simulink model "Sim_power_pedmap"  (R2025b)
settings: Solver=VariableStepAuto  StartTime=0.0  StopTime=15  RelTol=1e-3
undefined symbols (not defined in the file): LOCKED_FD_DAMP, LOCKED_FD_K, LOCKED_FD_OPT, M_DIFF_FD_TABLE, R_EFF_F_FD, R_EFF_R_FD, R_GEAR_FD
libraries: Solver_SF x1, simulink x1
settings Model: Creator=YNTM  LastModifiedBy=mayuan
settings RTWCC: GPUComputeCapability=3.5

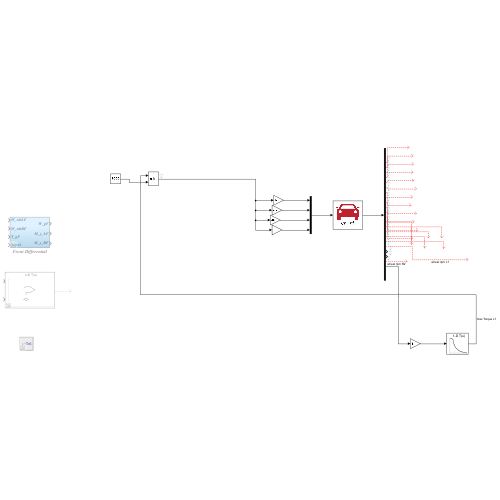
[thumbnail: Simulink's stored preview of the top-level diagram]
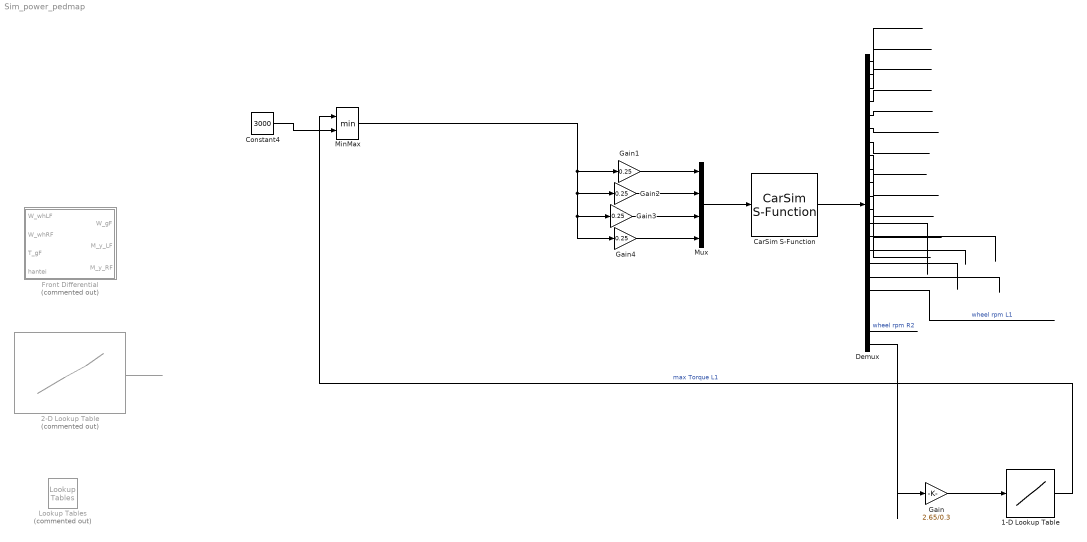
== system Sim_power_pedmap ==
  1-D Lookup Table : Lookup_n-D  NumberOfTableDimensions=1  BreakpointsForDimension1=[0, 50, 100, 150, 200, 250, 300, 350, 400, 450, 600].*3  Table=[3050, 3050, 2894.255, 1921.936, 1438.702, 1149.149, 956.489, 819.17, 717.149, 647.339, 477]  InternalRulePriority=Speed  RndMeth=Simplest
  2-D Lookup Table : Lookup_n-D  Commented=on  BreakpointsForDimension1=[0,5,15,20,25,30,40,50,60,70,80,90,100]  BreakpointsForDimension2=[0,7,10,20,30,40,50,60,70,80,100,120,140,160,180,200,220]  Table=|  InternalRulePriority=Speed  RndMeth=Simplest
      | [
      |     [0, 0, 0, 0, 0, 0, 0, 0, 0, 0, 0, 0, 0, 0, 0, 0, 0],
      |     [350, 350, 212, 104, 44, 22, 15, 15, 15, 15, 15, 15, 15, 15, 15, 15, 15],
      |     [765, 765, 641, 282, 149, 56, 100, 100, 100, 100, 100, 100, 100, 100, 100, 100, 100],
      |     [950, 950, 850, 621, 477, 354, 232, 200, 200, 200, 200, 200, 200, 200, 200, 200, 200],
      |     [1134, 1134, 1059, 959, 805, 652, 449, 300, 300, 300, 300, 300, 300, 300, 300, 300, 300],
      |     [1613, 1613, 1557, 1482, 1366, 1215, 1024, 846, 742, 656, 537, 463, 416, 398, 378, 362, 350],
      |     [2092, 2092, 2054, 2004, 1927, 1777, 1599, 1391, 1184, 1012, 774, 626, 532, 495, 455, 423, 400],
      |     [3049, 3049, 3049, 3049, 3049, 2902, 2749, 2482, 2068, 1724, 1247, 951, 763, 690, 610, 546, 500],
      |     [3752, 3752, 3752, 3752, 3751, 3629, 3484, 3235, 2850, 2524, 1978, 1598, 1329, 1173, 992, 867, 766],
      |     [4454, 4454, 4454, 4454, 4454, 4357, 4219, 3988, 3631, 3323, 2710, 2245, 1895, 1657, 1374, 1189, 1033],
      |     [5157, 5157, 5157, 5157, 5156, 5084, 4954, 4741, 4413, 4123, 3441, 2892, 2461, 2140, 1756, 1510, 1299],
      |     [5860, 5860, 5860, 5859, 5859, 5811, 5689, 5494, 5195, 4923, 4172, 3539, 3027, 2623, 2137, 1832, 1565],
      |     [6563, 6563, 6562, 6562, 6561, 6539, 6424, 6247, 5976, 5722, 4903, 4187, 3593, 3106, 2519, 2153, 1832],
      |     [7265, 7265, 7265, 7264, 7264, 7266, 7159, 7000, 6758, 6522, 5635, 4834, 4158, 3590, 2901, 2475, 2098]
      | ]
      settings: InputPortMap=u0,u1
  CarSim S-Function : Solver_SF/CarSim S-Function  Priority=1  SIMFILE=simfile.sim  Run_RTs=off  vs_state_ind=Run  StopMode_ind=Vehicle Model
  Constant4 : Constant  Value=3000
  Demux : Demux  Outputs=22
  "Front Differential " : Subsystem  Commented=on
  Gain : Gain  Gain=2.65/0.3
  Gain{1..4} (4 alike) : Gain  Gain=0.25
  Lookup Tables : simulink/Lookup Tables  Commented=on  SystemSampleTime=-1  VariantActivationTime=update diagram  EmptyChoice=off  PassThrough=off  PassThroughVariantControl=(default)  EmptyChoiceVariantControl=(default)  AllowFlexibleInterface=on  Latency=0  AutoFrameSizeCalculation=off
  MinMax : MinMax  Inputs=2
  Mux : Mux
  wires:
  MinMax/1 -> Gain4/1, Gain3/1, Gain2/1, Gain1/1
  Mux/1 -> CarSim S-Function/1
  CarSim S-Function/1 -> Demux/1
  Demux/1 -> ?
  Demux/2 -> ?
  Demux/3 -> ?
  Demux/4 -> ?
  Demux/5 -> ?
  Demux/6 -> ?
  Demux/7 -> ?
  Demux/8 -> ?
  Demux/9 -> ?
  Demux/10 -> ?
  Demux/11 -> ?
  Demux/12 -> ?
  Demux/13 -> ?
  Demux/14 -> ?
  Demux/15 -> ?
  Demux/16 -> ?
  Demux/17 -> ?
  2-D Lookup Table/1 -> ?
  Demux/18 -> ?  "wheel rpm L1"
  Demux/21 -> ?  "wheel rpm R2"
  1-D Lookup Table/1 -> MinMax/1  "max Torque L1"
  Constant4/1 -> MinMax/2
  Demux/22 -> Gain/1
  Gain/1 -> 1-D Lookup Table/1
  Gain1/1 -> Mux/1
  Gain2/1 -> Mux/2
  Gain3/1 -> Mux/3
  Gain4/1 -> Mux/4

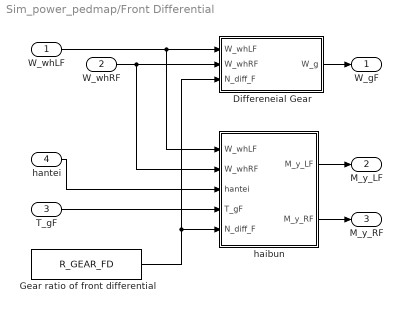
== system Sim_power_pedmap/Front Differential  ==
  W_whLF : Inport
  W_whRF : Inport  Port=2
  T_gF : Inport  Port=3
  hantei : Inport  Port=4
  Differeneial Gear : Subsystem
  Gear ratio of front differential : Constant  Value=R_GEAR_FD
  haibun : Subsystem
  W_gF : Outport
  M_y_LF : Outport  Port=2
  M_y_RF : Outport  Port=3
  wires:
  haibun/2(M_y_RF) -> M_y_RF/1
  haibun/1(M_y_LF) -> M_y_LF/1
  W_whRF/1 -> Differeneial Gear/2(W_whRF), haibun/2(W_whRF)
  W_whLF/1 -> Differeneial Gear/1(W_whLF), haibun/1(W_whLF)
  Gear ratio of front differential/1 -> haibun/5(N_diff_F), Differeneial Gear/3(N_diff_F)
  Differeneial Gear/1(W_g) -> W_gF/1
  T_gF/1 -> haibun/4(T_gF)
  hantei/1 -> haibun/3(hantei)

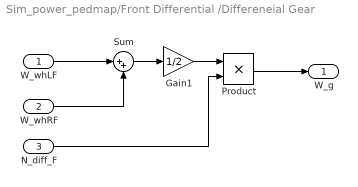
== system Sim_power_pedmap/Front Differential /Differeneial Gear ==
  W_whLF : Inport
  W_whRF : Inport  Port=2
  N_diff_F : Inport  Port=3
  Gain1 : Gain  Gain=1/2  SaturateOnIntegerOverflow=on  OutDataTypeStr=Inherit: Same as input  ParamDataTypeStr=Inherit: Same as input
  Product : Product  InputSameDT=on  SaturateOnIntegerOverflow=on  OutDataTypeStr=Inherit: Same as first input
  Sum : Sum  Inputs=|++  InputSameDT=on  SaturateOnIntegerOverflow=on  OutDataTypeStr=Inherit: Same as first input
  W_g : Outport
  wires:
  Product/1 -> W_g/1
  Gain1/1 -> Product/1
  W_whRF/1 -> Sum/2
  W_whLF/1 -> Sum/1
  N_diff_F/1 -> Product/2
  Sum/1 -> Gain1/1

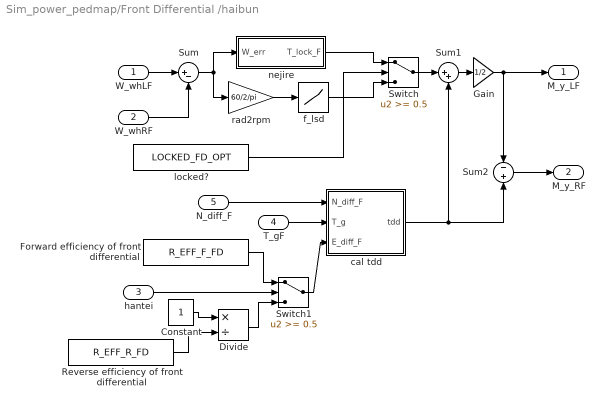
== system Sim_power_pedmap/Front Differential /haibun ==
  W_whLF : Inport
  W_whRF : Inport  Port=2
  hantei : Inport  Port=3
  T_gF : Inport  Port=4
  N_diff_F : Inport  Port=5
  Constant : Constant
  Divide : Product  Inputs=*/  InputSameDT=on  OutDataTypeStr=Inherit: Same as first input
  Forward efficiency of front differential : Constant  Value=R_EFF_F_FD
  Gain : Gain  Gain=1/2  SaturateOnIntegerOverflow=on  OutDataTypeStr=Inherit: Same as input  ParamDataTypeStr=Inherit: Same as input
  Reverse efficiency of front differential : Constant  Value=R_EFF_R_FD
  Sum : Sum  Inputs=|+-  InputSameDT=on  SaturateOnIntegerOverflow=on  OutDataTypeStr=Inherit: Same as first input
  Sum1 : Sum  Inputs=|++  InputSameDT=on  SaturateOnIntegerOverflow=on  OutDataTypeStr=Inherit: Same as first input
  Sum2 : Sum  Inputs=-|+  InputSameDT=on  SaturateOnIntegerOverflow=on  OutDataTypeStr=Inherit: Same as first input
  Switch : Switch  Threshold=0.5
  Switch1 : Switch  Threshold=0.5
  cal tdd : Subsystem
  f_lsd : Lookup  InputValues=M_DIFF_FD_TABLE(:,1)  Table=M_DIFF_FD_TABLE(:,2)
  locked? : Constant  Value=LOCKED_FD_OPT
  nejire : Subsystem
  rad2rpm : Gain  Gain=60/2/pi  SaturateOnIntegerOverflow=on  OutDataTypeStr=Inherit: Same as input  ParamDataTypeStr=Inherit: Same as input
  M_y_LF : Outport
  M_y_RF : Outport  Port=2
  wires:
  T_gF/1 -> cal tdd/2(T_g)
  hantei/1 -> Switch1/2
  Forward efficiency of front differential/1 -> Switch1/1
  Switch1/1 -> cal tdd/3(E_diff_F)
  W_whLF/1 -> Sum/1
  W_whRF/1 -> Sum/2
  cal tdd/1(tdd) -> Sum1/2, Sum2/2
  Sum2/1 -> M_y_RF/1
  N_diff_F/1 -> cal tdd/1(N_diff_F)
  nejire/1(T_lock_F) -> Switch/1
  Switch/1 -> Sum1/1
  rad2rpm/1 -> f_lsd/1
  Sum1/1 -> Gain/1
  Gain/1 -> M_y_LF/1, Sum2/1
  Sum/1 -> nejire/1(W_err), rad2rpm/1
  locked?/1 -> Switch/2
  f_lsd/1 -> Switch/3
  Constant/1 -> Divide/1
  Reverse efficiency of front differential/1 -> Divide/2
  Divide/1 -> Switch1/3

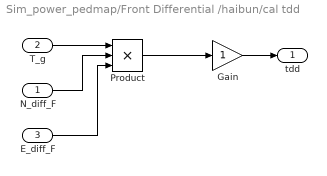
== system Sim_power_pedmap/Front Differential /haibun/cal tdd ==
  N_diff_F : Inport
  T_g : Inport  Port=2
  E_diff_F : Inport  Port=3
  Gain : Gain  SaturateOnIntegerOverflow=on  OutDataTypeStr=Inherit: Same as input  ParamDataTypeStr=Inherit: Same as input
  Product : Product  Inputs=3  InputSameDT=on  SaturateOnIntegerOverflow=on  OutDataTypeStr=Inherit: Same as first input
  tdd : Outport
  wires:
  Gain/1 -> tdd/1
  Product/1 -> Gain/1
  E_diff_F/1 -> Product/3
  N_diff_F/1 -> Product/2
  T_g/1 -> Product/1

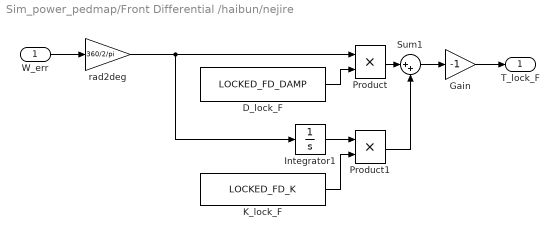
== system Sim_power_pedmap/Front Differential /haibun/nejire ==
  W_err : Inport
  D_lock_F : Constant  Value=LOCKED_FD_DAMP
  Gain : Gain  Gain=-1  SaturateOnIntegerOverflow=on  OutDataTypeStr=Inherit: Same as input  ParamDataTypeStr=Inherit: Same as input
  Integrator1 : Integrator
  K_lock_F : Constant  Value=LOCKED_FD_K
  Product : Product  InputSameDT=on  SaturateOnIntegerOverflow=on  OutDataTypeStr=Inherit: Same as first input
  Product1 : Product  InputSameDT=on  SaturateOnIntegerOverflow=on  OutDataTypeStr=Inherit: Same as first input
  Sum1 : Sum  Inputs=|++  InputSameDT=on  SaturateOnIntegerOverflow=on  OutDataTypeStr=Inherit: Same as first input
  rad2deg : Gain  Gain=360/2/pi  SaturateOnIntegerOverflow=on  OutDataTypeStr=Inherit: Same as input  ParamDataTypeStr=Inherit: Same as input
  T_lock_F : Outport
  wires:
  rad2deg/1 -> Integrator1/1, Product/1
  W_err/1 -> rad2deg/1
  Gain/1 -> T_lock_F/1
  Sum1/1 -> Gain/1
  D_lock_F/1 -> Product/2
  Integrator1/1 -> Product1/1
  K_lock_F/1 -> Product1/2
  Product1/1 -> Sum1/2
  Product/1 -> Sum1/1
